simulink model "Prelab1"  (R2018a)
settings: Solver=VariableStepAuto  StartTime=0.0  StopTime=10.0  RelTol=1e-3
libraries: simulink_extras x1, simulink x1
settings Model: Creator=mcjb87  LastModifiedBy=mcjb87

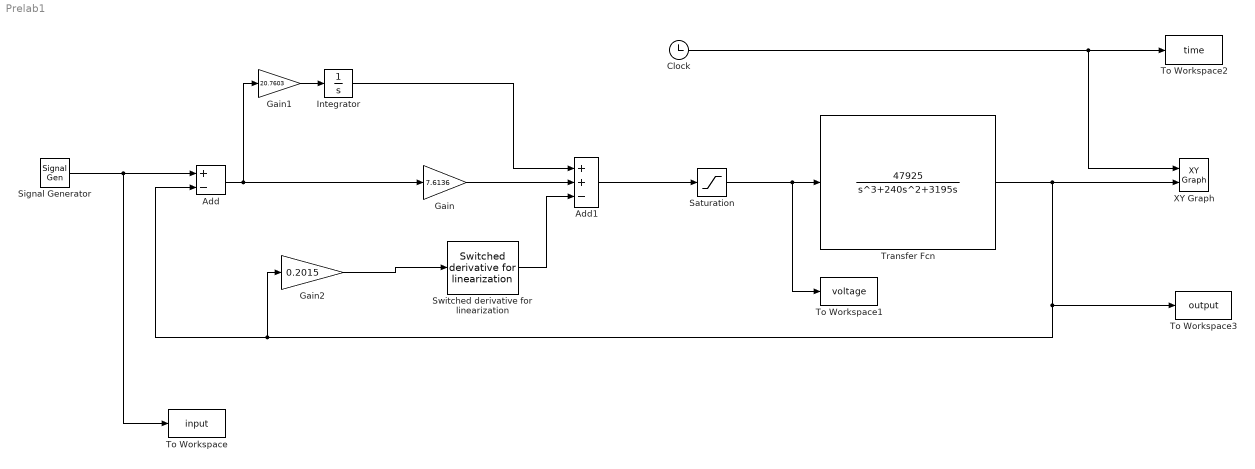
== system Prelab1 ==
  Add : Sum  Inputs=+-
  Add1 : Sum  Inputs=++-
  Clock : Clock
  Gain : Gain  Gain=7.6136
  Gain1 : Gain  Gain=20.7603
  Gain2 : Gain  Gain=0.2015
  Integrator : Integrator
  Saturation : Saturate  UpperLimit=+10  LowerLimit=-10
  Signal Generator : SignalGenerator  WaveForm=square  Amplitude=.6  Frequency=.6
  Switched derivative for linearization : simulink_extras/Linearization/Switched derivative for linearization  switchVal=0  derivConst=100
      settings: SourceProductName=Simulink  SourceProductBaseCode=SL
  To Workspace : ToWorkspace  VariableName=input  SaveFormat=Timeseries  SampleTime=-1
  To Workspace1 : ToWorkspace  VariableName=voltage  SaveFormat=Timeseries  SampleTime=-1
  To Workspace2 : ToWorkspace  VariableName=time  SaveFormat=Timeseries  SampleTime=-1
  To Workspace3 : ToWorkspace  VariableName=output  SaveFormat=Timeseries  SampleTime=-1
  Transfer Fcn : TransferFcn  Numerator=47925  Denominator=[1 240 3195 0]
  XY Graph : simulink/Sinks/XY Graph  xmin=0  xmax=10  ymin=-1.5  ymax=1.5  st=-1
  wires:
  Signal Generator/1 -> To Workspace/1, Add/1
  Add/1 -> Gain1/1, Gain/1
  Gain/1 -> Add1/2
  Add1/1 -> Saturation/1
  Saturation/1 -> To Workspace1/1, Transfer Fcn/1
  Gain1/1 -> Integrator/1
  Integrator/1 -> Add1/1
  Gain2/1 -> Switched derivative for linearization/1
  Switched derivative for linearization/1 -> Add1/3
  Transfer Fcn/1 -> To Workspace3/1, Gain2/1, Add/2, XY Graph/2
  Clock/1 -> XY Graph/1, To Workspace2/1
